simulink model "models"  (R2014b)
settings: Solver=VariableStepAuto  StartTime=0.0  StopTime=inf  RelTol=1e-3
values from neighbouring files (symbols this model uses):
  A = str2double(b)    [MatlabClient.m]
  tc = now    [MatlabClient.m]
  temp = t    [MatlabClient.m]
  tl = 0    [MatlabClient.m]
  tx = now    [MatlabClient.m]
settings Model: Creator=rohit  LastModifiedBy=student
settings DataIOCC: SaveFormat=Dataset
settings OptimizationCC: UseDivisionForNetSlopeComputation=off  SimCompilerOptimization=off
settings DebuggingCC: SolverPrmCheckMsg=none  FrameProcessingCompatibilityMsg=error  AllowSymbolicDim=off
settings HardwareCC: ProdBitPerPointer=64  ProdLargestAtomicFloat=Float  ProdIntDivRoundTo=Zero  ProdEndianess=LittleEndian  ProdWordSize=64  ProdHWDeviceType=Intel->x86-64 (Windows64)
settings RTWCC: RTWCompilerOptimization=off
settings GRTTargetCC: GeneratePreprocessorConditionals=Use local settings
settings ConfigComp: CovMetricSettings=dw  CovHtmlReporting=on  CovSaveCumulativeToWorkspaceVar=on  CovSaveSingleToWorkspaceVar=on  CovExternalEMLEnable=off

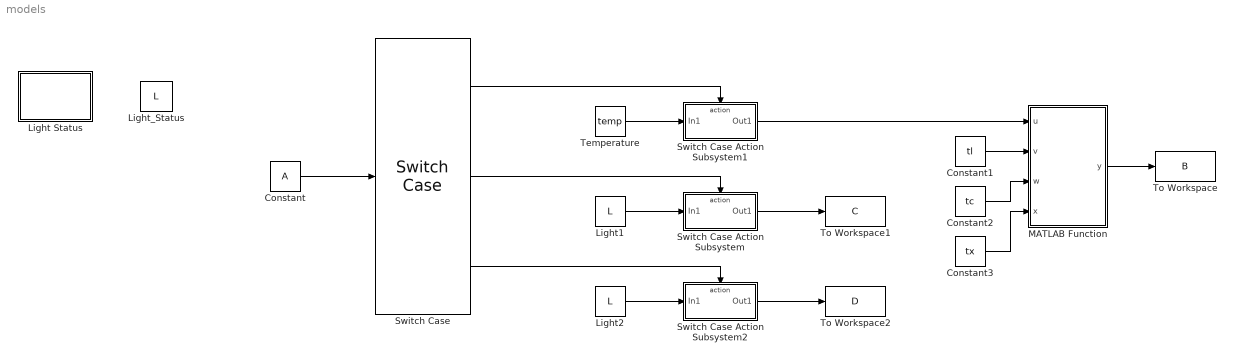
== system models ==
  Constant : Constant  Value=A
  Constant1 : Constant  Value=tl
  Constant2 : Constant  Value=tc
  Constant3 : Constant  Value=tx
  Light Status : MATLAB Function  TreatAsAtomicUnit=on
  Light1 : DataStoreRead  DataStoreName=L
  Light2 : DataStoreRead  DataStoreName=L
  Light_Status : DataStoreMemory  DataStoreName=L  ReadBeforeWriteMsg=warning  WriteAfterWriteMsg=warning  WriteAfterReadMsg=warning  OutDataTypeStr=double
      settings: RTWStateStorageClass=ExportedGlobal
  MATLAB Function : MATLAB Function  TreatAsAtomicUnit=on
  Switch Case : SwitchCase  CaseConditions={1,2,3}  ShowDefaultCase=off
  Switch Case Action Subsystem : Subsystem  TreatAsAtomicUnit=on
  Switch Case Action Subsystem1 : Subsystem  TreatAsAtomicUnit=on
  Switch Case Action Subsystem2 : Subsystem  TreatAsAtomicUnit=on
  Temperature : Constant  Value=temp
  To Workspace : ToWorkspace  VariableName=B  SaveFormat=Timeseries  SampleTime=-1
  To Workspace1 : ToWorkspace  VariableName=C  SaveFormat=Timeseries  SampleTime=-1
  To Workspace2 : ToWorkspace  VariableName=D  SaveFormat=Timeseries  SampleTime=-1
  wires:
  Switch Case/2 -> Switch Case Action Subsystem/Action
  Switch Case Action Subsystem1/1(Out1) -> MATLAB Function/1(u)
  Light1/1 -> Switch Case Action Subsystem/1(In1)
  Constant/1 -> Switch Case/1
  Temperature/1 -> Switch Case Action Subsystem1/1(In1)
  Switch Case Action Subsystem2/1(Out1) -> To Workspace2/1
  Light2/1 -> Switch Case Action Subsystem2/1(In1)
  Switch Case/3 -> Switch Case Action Subsystem2/Action
  Switch Case/1 -> Switch Case Action Subsystem1/Action
  Switch Case Action Subsystem/1(Out1) -> To Workspace1/1
  MATLAB Function/1(y) -> To Workspace/1
  Constant1/1 -> MATLAB Function/2(v)
  Constant2/1 -> MATLAB Function/3(w)
  Constant3/1 -> MATLAB Function/4(x)

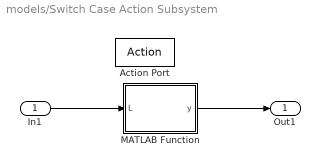
== system models/Switch Case Action Subsystem ==
  In1 : Inport
  Action Port : ActionPort  ActionType=case
  MATLAB Function : MATLAB Function  TreatAsAtomicUnit=on
  Out1 : Outport
  wires:
  In1/1 -> MATLAB Function/1(L)
  MATLAB Function/1(y) -> Out1/1

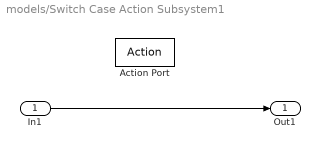
== system models/Switch Case Action Subsystem1 ==
  In1 : Inport
  Action Port : ActionPort  ActionType=case
  Out1 : Outport
  wires:
  In1/1 -> Out1/1

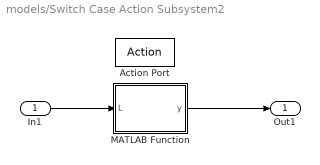
== system models/Switch Case Action Subsystem2 ==
  In1 : Inport
  Action Port : ActionPort  ActionType=case
  MATLAB Function : MATLAB Function  TreatAsAtomicUnit=on
  Out1 : Outport
  wires:
  In1/1 -> MATLAB Function/1(L)
  MATLAB Function/1(y) -> Out1/1

== matlab function models/MATLAB Function ==
  data: u input; y output; v input; w input; x input
function y = fcn(u, v, w, x)
%#codegen
if (v == 0 && x == 0)
    y = u;
elseif (x == 0 && v ~= 0)
    y = u + (w - v)*10000;
else
    y = u - (w - x)*10000;
end

== matlab function models/Light Status ==
  data: L data_store_memory
function fcn
%#codegen
global L;
L = 3;

== matlab function models/Switch Case Action Subsystem/MATLAB Function ==
  data: L input; y output
function y = fcn(L)
%#codegen
if L == 3
    L = 2;
end
y = L;

== matlab function models/Switch Case Action Subsystem2/MATLAB Function ==
  data: L input; y output
function y = fcn(L)
%#codegen
if L == 2
    L = 3;
end
y = L;
